simulink model "SecRwLtStFtrstCtrl"  (R2018b)
settings: Solver=FixedStepDiscrete  StartTime=0.0  StopTime=10.0  FixedStep=0.01  RelTol=1e-3
undefined symbols (not defined in the file or in its folder): KeSMSuMdMotFinshdTm_Val, KeSMSuMdRetryTm1_Val, KeSMSuModeReqDurgTm_Val, KeSMSwSecRwLtStFtrstEnTrigBitMask_Val
libraries: StCtrlLib x1
settings Model: Creator=sn2xws  LastModifiedBy=sn2xws
settings DataIOCC: SaveFormat=StructureWithTime
settings OptimizationCC: DefaultParameterBehavior=Inlined  EnhancedBackFolding=on  PassReuseOutputArgsAs=Individual arguments  ZeroExternalMemoryAtStartup=off  ZeroInternalMemoryAtStartup=off  OptimizeBlockOrder=speed  DifferentSizesBufferReuse=on  OptimizationCustomize=off
settings DebuggingCC: ParameterTunabilityLossMsg=error
settings ModelReferenceCC: ModelReferenceNumInstancesAllowed=Single
settings SFSimCC: MATLABDynamicMemAlloc=off
settings RTWCC: SystemTargetFile=autosar.tlc  GenCodeOnly=on  TemplateMakefile=ert_default_tmf  Description=AUTOSAR  GenerateReport=on  IncludeHyperlinkInReport=on  LaunchReport=on  GenerateTraceInfo=on  GenerateTraceReport=on  GenerateTraceReportSl=on  GenerateTraceReportSf=on  GenerateTraceReportEml=on
settings CodeAppCC: ForceParamTrailComments=on  IgnoreCustomStorageClasses=off  OperatorAnnotations=on  SimulinkDataObjDesc=on  SFDataObjDesc=on  InsertBlockDesc=on
settings STFCustomTargetCC: TargetLangStandard=C99 (ISO)  MultiwordLength=256  ParMdlRefBuildCompliant=on  CompOptLevelCompliant=on  IncludeMdlTerminateFcn=off  CombineOutputUpdateFcns=on  SuppressErrorStatus=on  ERTCustomFileBanners=on  SupportNonFinite=off  SupportComplex=off  SupportContinuousTime=off  SupportNonInlinedSFcns=off  RemoveResetFunc=on  MATLABClassNameForMDSCustomization=Simulink.SoftwareTarget.ERTCustomization  AutosarCompliant=on  UseToolchainInfoCompliant=on  LookupTableObjectStructAxisOrder=2,1,3,4,...  LUTObjectStructOrderEvenSpacing=Size,Table,Breakpoints  SystemTargetFile=autosar.tlc
settings ERTTargetCC: TargetLangStandard=C99 (ISO)  ConcurrentExecutionCompliant=off  IncludeMdlTerminateFcn=off  SuppressErrorStatus=on  SupportNonFinite=off  SupportComplex=off  ModelStepFunctionPrototypeControlCompliant=off  CPPClassGenCompliant=off  AutosarCompliant=on  LookupTableObjectStructAxisOrder=2,1,3,4,...  LUTObjectStructOrderEvenSpacing=Size,Table,Breakpoints  InlinedParameterPlacement=NonHierarchical  ERTCustomFileTemplate=example_file_process.tlc  ERTFilePackagingFormat=Compact

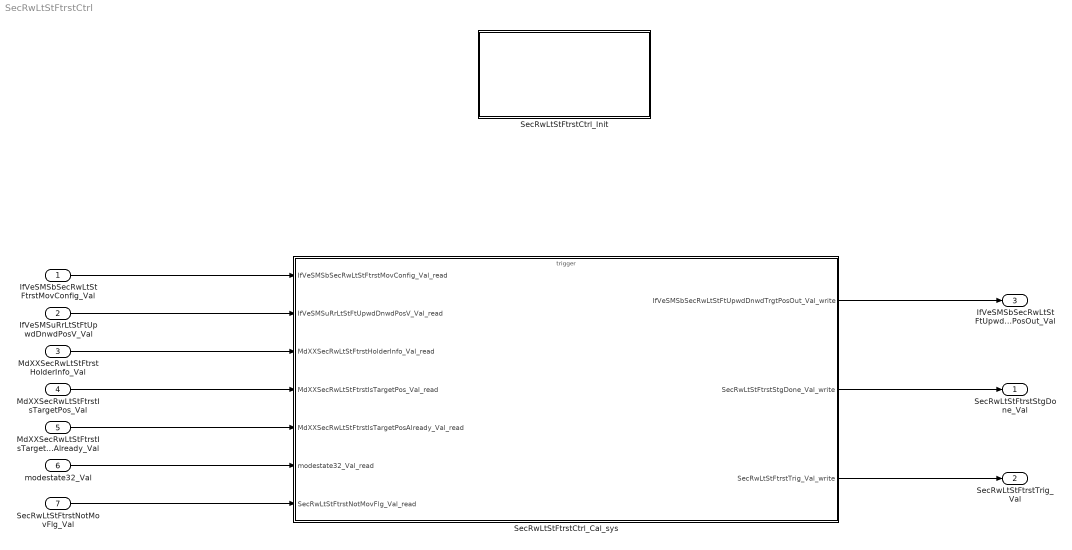
== system SecRwLtStFtrstCtrl ==
  IfVeSMSbSecRwLtStFtrstMovConfig_Val : Inport  OutDataTypeStr=boolean  PortDimensions=1
  IfVeSMSuRrLtStFtUpwdDnwdPosV_Val : Inport  Port=2  OutDataTypeStr=boolean  PortDimensions=1
  MdXXSecRwLtStFtrstHolderInfo_Val : Inport  Port=3  OutDataTypeStr=uint32  PortDimensions=1
  MdXXSecRwLtStFtrstIsTargetPos_Val : Inport  Port=4  OutDataTypeStr=uint32  PortDimensions=1
  MdXXSecRwLtStFtrstIsTargetPosAlready_Val : Inport  Port=5  OutDataTypeStr=uint32  PortDimensions=1
  modestate32_Val : Inport  Port=6  OutDataTypeStr=uint32  PortDimensions=1
  SecRwLtStFtrstNotMovFlg_Val : Inport  Port=7  OutDataTypeStr=boolean  PortDimensions=1
  SecRwLtStFtrstCtrl_Cal_sys : Subsystem
  SecRwLtStFtrstCtrl_Init : Subsystem
  SecRwLtStFtrstStgDone_Val : Outport  OutDataTypeStr=boolean  PortDimensions=1
  SecRwLtStFtrstTrig_Val : Outport  Port=2  OutDataTypeStr=boolean  PortDimensions=1
  IfVeSMSbSecRwLtStFtUpwdDnwdTrgtPosOut_Val : Outport  Port=3  OutDataTypeStr=boolean  PortDimensions=1
  wires:
  SecRwLtStFtrstCtrl_Cal_sys/1(IfVeSMSbSecRwLtStFtUpwdDnwdTrgtPosOut_Val_write) -> IfVeSMSbSecRwLtStFtUpwdDnwdTrgtPosOut_Val/1
  SecRwLtStFtrstCtrl_Cal_sys/2(SecRwLtStFtrstStgDone_Val_write) -> SecRwLtStFtrstStgDone_Val/1
  SecRwLtStFtrstCtrl_Cal_sys/3(SecRwLtStFtrstTrig_Val_write) -> SecRwLtStFtrstTrig_Val/1
  SecRwLtStFtrstNotMovFlg_Val/1 -> SecRwLtStFtrstCtrl_Cal_sys/7(SecRwLtStFtrstNotMovFlg_Val_read)
  modestate32_Val/1 -> SecRwLtStFtrstCtrl_Cal_sys/6(modestate32_Val_read)
  MdXXSecRwLtStFtrstIsTargetPosAlready_Val/1 -> SecRwLtStFtrstCtrl_Cal_sys/5(MdXXSecRwLtStFtrstIsTargetPosAlready_Val_read)
  MdXXSecRwLtStFtrstIsTargetPos_Val/1 -> SecRwLtStFtrstCtrl_Cal_sys/4(MdXXSecRwLtStFtrstIsTargetPos_Val_read)
  MdXXSecRwLtStFtrstHolderInfo_Val/1 -> SecRwLtStFtrstCtrl_Cal_sys/3(MdXXSecRwLtStFtrstHolderInfo_Val_read)
  IfVeSMSuRrLtStFtUpwdDnwdPosV_Val/1 -> SecRwLtStFtrstCtrl_Cal_sys/2(IfVeSMSuRrLtStFtUpwdDnwdPosV_Val_read)
  IfVeSMSbSecRwLtStFtrstMovConfig_Val/1 -> SecRwLtStFtrstCtrl_Cal_sys/1(IfVeSMSbSecRwLtStFtrstMovConfig_Val_read)

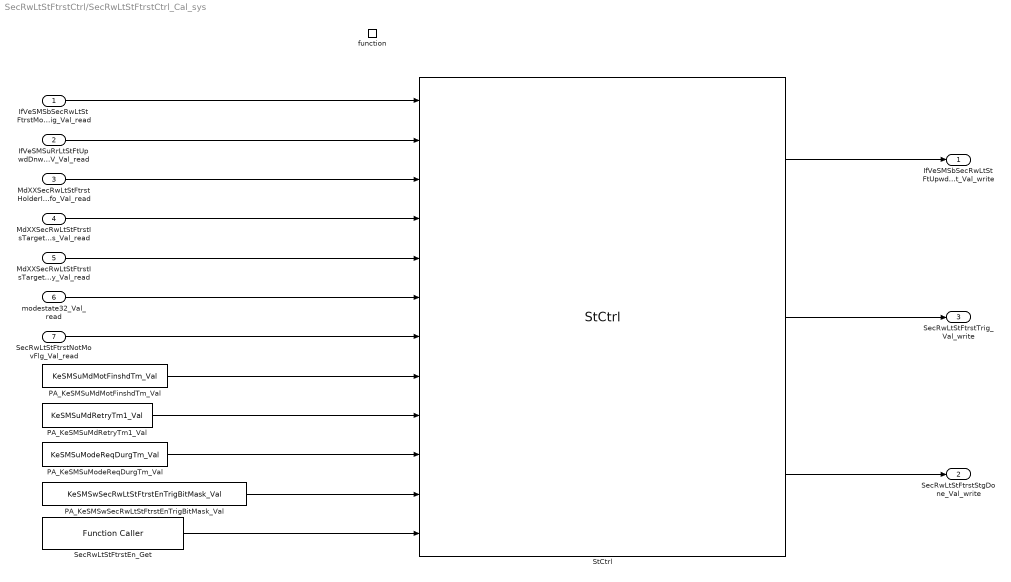
== system SecRwLtStFtrstCtrl/SecRwLtStFtrstCtrl_Cal_sys ==
  IfVeSMSbSecRwLtStFtrstMovConfig_Val_read : Inport
  IfVeSMSuRrLtStFtUpwdDnwdPosV_Val_read : Inport  Port=2
  MdXXSecRwLtStFtrstHolderInfo_Val_read : Inport  Port=3
  MdXXSecRwLtStFtrstIsTargetPos_Val_read : Inport  Port=4
  MdXXSecRwLtStFtrstIsTargetPosAlready_Val_read : Inport  Port=5
  modestate32_Val_read : Inport  Port=6
  SecRwLtStFtrstNotMovFlg_Val_read : Inport  Port=7
  function : TriggerPort  TriggerType=function-call  IsSimulinkFunction=on  FunctionName=SecRwLtStFtrstCtrl_Cal  VariantControl=(inherit)
  PA_KeSMSuMdMotFinshdTm_Val : Constant  Value=KeSMSuMdMotFinshdTm_Val
  PA_KeSMSuMdRetryTm1_Val : Constant  Value=KeSMSuMdRetryTm1_Val
  PA_KeSMSuModeReqDurgTm_Val : Constant  Value=KeSMSuModeReqDurgTm_Val
  PA_KeSMSwSecRwLtStFtrstEnTrigBitMask_Val : Constant  Value=KeSMSwSecRwLtStFtrstEnTrigBitMask_Val
  SecRwLtStFtrstEn_Get : FunctionCaller  FunctionPrototype=data = SecRwLtStFtrstEn_Get()  OutputArgumentSpecifications=uint32(1)
  StCtrl : StCtrlLib/StCtrl  SystemSampleTime=-1
  IfVeSMSbSecRwLtStFtUpwdDnwdTrgtPosOut_Val_write : Outport
      settings: EnsureOutportIsVirtual=on
  SecRwLtStFtrstStgDone_Val_write : Outport  Port=2
      settings: EnsureOutportIsVirtual=on
  SecRwLtStFtrstTrig_Val_write : Outport  Port=3
      settings: EnsureOutportIsVirtual=on
  wires:
  StCtrl/1 -> IfVeSMSbSecRwLtStFtUpwdDnwdTrgtPosOut_Val_write/1
  StCtrl/2 -> SecRwLtStFtrstTrig_Val_write/1
  StCtrl/3 -> SecRwLtStFtrstStgDone_Val_write/1
  PA_KeSMSwSecRwLtStFtrstEnTrigBitMask_Val/1 -> StCtrl/11
  PA_KeSMSuMdMotFinshdTm_Val/1 -> StCtrl/8
  PA_KeSMSuModeReqDurgTm_Val/1 -> StCtrl/10
  SecRwLtStFtrstEn_Get/1 -> StCtrl/12
  PA_KeSMSuMdRetryTm1_Val/1 -> StCtrl/9
  IfVeSMSbSecRwLtStFtrstMovConfig_Val_read/1 -> StCtrl/1
  IfVeSMSuRrLtStFtUpwdDnwdPosV_Val_read/1 -> StCtrl/2
  MdXXSecRwLtStFtrstHolderInfo_Val_read/1 -> StCtrl/3
  MdXXSecRwLtStFtrstIsTargetPos_Val_read/1 -> StCtrl/4
  MdXXSecRwLtStFtrstIsTargetPosAlready_Val_read/1 -> StCtrl/5
  modestate32_Val_read/1 -> StCtrl/6
  SecRwLtStFtrstNotMovFlg_Val_read/1 -> StCtrl/7

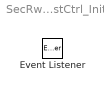
== system SecRwLtStFtrstCtrl/SecRwLtStFtrstCtrl_Init ==
  Event Listener : EventListener  EventName=reset
